simulink model "CoAS_RlsCmpn"  (R2016b)
settings: configuration reference "CodeGenConfigSet" (kept outside this file)
values from neighbouring files (symbols this model uses):
  CoAS_stEGRVlv_C = Calibration.Parameter    [init_CoAS_RlsCmpn.m]
  CoAS_stThrVlv_C = Calibration.Parameter    [init_CoAS_RlsCmpn.m]
settings Model: Creator=Wollf  LastModifiedBy=lenovo
settings ConfigSetRef: SourceLocation=Base Workspace

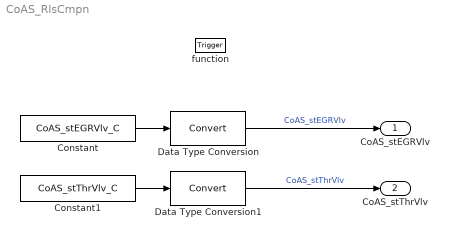
== system CoAS_RlsCmpn ==
  function : TriggerPort  TriggerType=function-call  VariantControl=Variant
  Constant : Constant  Value=CoAS_stEGRVlv_C
  Constant1 : Constant  Value=CoAS_stThrVlv_C
  Data Type Conversion : DataTypeConversion
  Data Type Conversion1 : DataTypeConversion
  CoAS_stEGRVlv : Outport  Description="State  of EGR control enable"  OutMin=0  OutMax=255  OutDataTypeStr=State_uint8
  CoAS_stThrVlv : Outport  Description="State  of TVA control enable"  Port=2  OutMin=0  OutMax=255  OutDataTypeStr=State_uint8
  wires:
  Constant/1 -> Data Type Conversion/1
  Data Type Conversion/1 -> CoAS_stEGRVlv/1  "CoAS_stEGRVlv"
  Constant1/1 -> Data Type Conversion1/1
  Data Type Conversion1/1 -> CoAS_stThrVlv/1  "CoAS_stThrVlv"
